simulink model "ES005A_TmplMonr"  (R2013b)
settings: Solver=FixedStepDiscrete  SolverMode=SingleTasking  StartTime=0.0  StopTime=1  FixedStep=0.002  RelTol=1e-3
undefined symbols (not defined in the file): ELECGLBPRM_STRTUPSTDI_CNT_U08, ELECGLBPRM_STRTUPSTTMPLMONININTESTSTRT_CNT_U08, IninFlt, RtFlt, SpiConf_SpiChannel_TmplMonrCh1, SpiConf_SpiChannel_TmplMonrCh2, SpiConf_SpiChannel_TmplMonrCh3, SpiConf_SpiSequence_TmplMonrSeq1, SpiConf_SpiSequence_TmplMonrSeq2, SpiConf_SpiSequence_TmplMonrSeq3, STD_HIGH, STD_LOW, TMPLMONRCFGREG1READVAL_CNT_U16, TMPLMONRCFGREG1WRVAL_CNT_U16, TMPLMONRSTSREG2READVAL_CNT_U16, TMPLMONRWDGMODKEYWORD1_CNT_U16, TMPLMONRWDGMODKEYWORD2_CNT_U16, TMPLMONRWDGMODKEYWORD3_CNT_U16, TrigReg1
libraries: simulink x12
(part 3 of 4)

== system ES005A_TmplMonr/TmplMonr/TmplMonrPer1/TMF Init Test/21/CopyRight1 ==

== system ES005A_TmplMonr/TmplMonr/TmplMonrPer1/TMF Init Test/21/Edge//Valid Cnts are NOT Correct ==
  note: NTCNR_0X040
      | Parameters:
      |     1 = 0000 0001 = Bit 0 = Fault Occured Between TmplMonrInitCntr =  10 ~ 11
      |     2 = 0000 0010 = Bit 1 = Fault Occured Between TmplMonrInitCntr = 13 (AND Gate Fault)
      |     4 = 0000 0100 = Bit 2 = Fault Occured Between TmplMonrInitCntr = 15 ~ 16
      |     8 = 0000 1000 = Bit 3 = Fault Occured at TmplMonrInitCntr            = 18  (POE Fault)
      |   16 = 0001 0000 = Bit 4 = Fault Occured at TmplMonrInitCntr            = 19 (WD_STATE Fault)
      |   32 = 0010 0000 = Bit 5 = Fault Occured at TmplMonrInitCntr            = 21 (Edge/Valid Write Fault)
      |   64 = 0100 0000 = Bit 6 = Fault Occured at TmplMonrInitCntr            = 53 (POE + Non-WD Fault)
      | 128 = 1000 0000 = Bit 7 = Fault Occured at TmplMonrInitCntr            = 53 (POE + WD Fault)
  Action Port : ActionPort  ActionType=then
  Bitwise Operator2 : simulink/Logic and Bit Operations/Bitwise Operator  logicop=OR  UseBitMask=off  NumInputPorts=2  BitMask=bin2dec('00001111')  BitMaskRealWorld=Stored Integer
  CopyRight1 : Subsystem  Description=|  mask(Copyright Information){none=on}
      | Copyright info block.                                               
      |                                                                     
      | Place copyright information at the top of every subsystem in design.
      mask prompts: none "No parameters"
      mask help: Place copyright information at the top of every subsystem in design.
      mask Display:
      | NxtrConf = 'Nexteer Confidential';
      | 
      | sys = bdroot; %handle for the current model ("system")
      | first = get_param(sys,'Created');
      | first = first(end-3:end);  %year is last four digits
      | 
      | last = get_param(sys,'LastModifiedDate');
      | if isempty(last)
      |     last = datestr(now,'yyyy');
      | else
      |     last = last(end-3:end);
      | end
      | 
      | if strcmp(first,last)
      |     fprintf('%s -- Copyright %s Nexteer',NxtrConf,first)
      | else
      |     fprintf('%s -- %s%s- %s Nexteer',NxtrConf,char(169),first,last)
      | end
  Data Store Read3 : DataStoreRead  DataStoreName=TmplMonrNtc40PrmByte  DataStoreElements=TmplMonrNtc40PrmByte
  Data Store Write1 : DataStoreWrite  DataStoreName=TmplMonrNtc40PrmByte
  NtcStInfo : Constant  Value=32  OutDataTypeStr=uint8
  wires:
  Bitwise Operator2/1 -> Data Store Write1/1
  Data Store Read3/1 -> Bitwise Operator2/1
  NtcStInfo/1 -> Bitwise Operator2/2

== system ES005A_TmplMonr/TmplMonr/TmplMonrPer1/TMF Init Test/21/Spi_ReadIB ==
  note: Read Buffer - Simulation Purpose Only
      |
      |
      |
      |                            00001011
  Channel : Inport
  Constant1 : Constant  Value=11  OutDataTypeStr=uint16
  CopyRight1 : Subsystem  Description=|  mask(Copyright Information){none=on}
      | Copyright info block.                                               
      |                                                                     
      | Place copyright information at the top of every subsystem in design.
      mask prompts: none "No parameters"
      mask help: Place copyright information at the top of every subsystem in design.
      mask Display:
      | NxtrConf = 'Nexteer Confidential';
      | 
      | sys = bdroot; %handle for the current model ("system")
      | first = get_param(sys,'Created');
      | first = first(end-3:end);  %year is last four digits
      | 
      | last = get_param(sys,'LastModifiedDate');
      | if isempty(last)
      |     last = datestr(now,'yyyy');
      | else
      |     last = last(end-3:end);
      | end
      | 
      | if strcmp(first,last)
      |     fprintf('%s -- Copyright %s Nexteer',NxtrConf,first)
      | else
      |     fprintf('%s -- %s%s- %s Nexteer',NxtrConf,char(169),first,last)
      | end
  Terminator : Terminator
  Rx : Outport
  wires:
  Constant1/1 -> Rx/1
  Channel/1 -> Terminator/1

== system ES005A_TmplMonr/TmplMonr/TmplMonrPer1/TMF Init Test/22-52/CopyRight1 ==

== system ES005A_TmplMonr/TmplMonr/TmplMonrPer1/TMF Init Test/53/CopyRight1 ==

== system ES005A_TmplMonr/TmplMonr/TmplMonrPer1/TMF Init Test/53/Fault Condition - WD Run Fault ==
  Action Port : ActionPort  ActionType=else
  CopyRight1 : Subsystem  Description=|  mask(Copyright Information){none=on}
      | Copyright info block.                                               
      |                                                                     
      | Place copyright information at the top of every subsystem in design.
      mask prompts: none "No parameters"
      mask help: Place copyright information at the top of every subsystem in design.
      mask Display:
      | NxtrConf = 'Nexteer Confidential';
      | 
      | sys = bdroot; %handle for the current model ("system")
      | first = get_param(sys,'Created');
      | first = first(end-3:end);  %year is last four digits
      | 
      | last = get_param(sys,'LastModifiedDate');
      | if isempty(last)
      |     last = datestr(now,'yyyy');
      | else
      |     last = last(end-3:end);
      | end
      | 
      | if strcmp(first,last)
      |     fprintf('%s -- Copyright %s Nexteer',NxtrConf,first)
      | else
      |     fprintf('%s -- %s%s- %s Nexteer',NxtrConf,char(169),first,last)
      | end
  Data Store Read1 : DataStoreRead  DataStoreName=TmplMonrSpiReadWrOrderFlg1
  If : If  IfExpression=u1 == 0
  Merge1 : Merge
  Merge2 : Merge
  "TmplMonrSpiReadWrOrderFlg1 = 0 (Read Cmd) " : Subsystem
  TmplMonrSpiReadWrOrderFlg1 = 1 (Read Buffer) : Subsystem
  TmplMonrInitCntr : Outport
  TmplMonrIninTestCmpl : Outport  Port=2
  wires:
  If/1 -> "TmplMonrSpiReadWrOrderFlg1 = 0 (Read Cmd) "/Action
  If/2 -> TmplMonrSpiReadWrOrderFlg1 = 1 (Read Buffer)/Action
  Data Store Read1/1 -> If/1
  Merge1/1 -> TmplMonrInitCntr/1
  "TmplMonrSpiReadWrOrderFlg1 = 0 (Read Cmd) "/1(TmplMonrIninCntr) -> Merge1/1
  TmplMonrSpiReadWrOrderFlg1 = 1 (Read Buffer)/1(TmplMonrIninCntr) -> Merge1/2
  "TmplMonrSpiReadWrOrderFlg1 = 0 (Read Cmd) "/2(TmplMonrIninTestCmpl) -> Merge2/1
  TmplMonrSpiReadWrOrderFlg1 = 1 (Read Buffer)/2(TmplMonrIninTestCmpl) -> Merge2/2
  Merge2/1 -> TmplMonrIninTestCmpl/1

== system ES005A_TmplMonr/TmplMonr/TmplMonrPer1/TMF Init Test/53/IoHwAb_GetGpioPwrOutpEnaFb ==
  CopyRight1 : Subsystem  Description=|  mask(Copyright Information){none=on}
      | Copyright info block.                                               
      |                                                                     
      | Place copyright information at the top of every subsystem in design.
      mask prompts: none "No parameters"
      mask help: Place copyright information at the top of every subsystem in design.
      mask Display:
      | NxtrConf = 'Nexteer Confidential';
      | 
      | sys = bdroot; %handle for the current model ("system")
      | first = get_param(sys,'Created');
      | first = first(end-3:end);  %year is last four digits
      | 
      | last = get_param(sys,'LastModifiedDate');
      | if isempty(last)
      |     last = datestr(now,'yyyy');
      | else
      |     last = last(end-3:end);
      | end
      | 
      | if strcmp(first,last)
      |     fprintf('%s -- Copyright %s Nexteer',NxtrConf,first)
      | else
      |     fprintf('%s -- %s%s- %s Nexteer',NxtrConf,char(169),first,last)
      | end
  Ground : Ground
  PinSt : Outport
  wires:
  Ground/1 -> PinSt/1

== system ES005A_TmplMonr/TmplMonr/TmplMonrPer1/TMF Init Test/53/Normal Condition ==
  Action Port : ActionPort  ActionType=then
  Constant1 : Constant  OutDataTypeStr=boolean
  Constant2 : Constant  OutDataTypeStr=uint8
  Constant3 : Constant  Value=0  OutDataTypeStr=boolean
  Constant4 : Constant  OutDataTypeStr=boolean
  CopyRight1 : Subsystem  Description=|  mask(Copyright Information){none=on}
      | Copyright info block.                                               
      |                                                                     
      | Place copyright information at the top of every subsystem in design.
      mask prompts: none "No parameters"
      mask help: Place copyright information at the top of every subsystem in design.
      mask Display:
      | NxtrConf = 'Nexteer Confidential';
      | 
      | sys = bdroot; %handle for the current model ("system")
      | first = get_param(sys,'Created');
      | first = first(end-3:end);  %year is last four digits
      | 
      | last = get_param(sys,'LastModifiedDate');
      | if isempty(last)
      |     last = datestr(now,'yyyy');
      | else
      |     last = last(end-3:end);
      | end
      | 
      | if strcmp(first,last)
      |     fprintf('%s -- Copyright %s Nexteer',NxtrConf,first)
      | else
      |     fprintf('%s -- %s%s- %s Nexteer',NxtrConf,char(169),first,last)
      | end
  Data Store Write : DataStoreWrite  DataStoreName=TmplMonrSpiReadWrOrderFlg1
  Data Store Write2 : DataStoreWrite  DataStoreName=TmplMonrIninTestCmplFlg
      settings: AttributesFormatString=%<Name>
  TmplMonrIninCntr : Outport
  TmplMonrIninTestCmpl : Outport  Port=2
  wires:
  Constant2/1 -> TmplMonrIninCntr/1
  Constant1/1 -> TmplMonrIninTestCmpl/1
  Constant3/1 -> Data Store Write/1
  Constant4/1 -> Data Store Write2/1

== system ES005A_TmplMonr/TmplMonr/TmplMonrPer1/TMF Init Test/53/Set NTC 0x040 Note: Run last ==
  note: NTCNR_0X040
      | Parameters:
      |     1 = 0000 0001 = Bit 0 = Fault Occured Between TmplMonrInitCntr =  10 ~ 11
      |     2 = 0000 0010 = Bit 1 = Fault Occured Between TmplMonrInitCntr = 13 (AND Gate Fault)
      |     4 = 0000 0100 = Bit 2 = Fault Occured Between TmplMonrInitCntr = 15 ~ 16
      |     8 = 0000 1000 = Bit 3 = Fault Occured at TmplMonrInitCntr            = 18  (POE Fault)
      |   16 = 0001 0000 = Bit 4 = Fault Occured at TmplMonrInitCntr            = 19 (WD_STATE Fault)
      |   32 = 0010 0000 = Bit 5 = Fault Occured at TmplMonrInitCntr            = 21 (Edge/Valid Write Fault)
      |   64 = 0100 0000 = Bit 6 = Fault Occured at TmplMonrInitCntr            = 53 (POE + Non-WD Fault)
      | 128 = 1000 0000 = Bit 7 = Fault Occured at TmplMonrInitCntr            = 53 (POE + WD Fault)
  Data Store Read2 : DataStoreRead  DataStoreName=TmplMonrNtc40PrmByte  DataStoreElements=TmplMonrNtc40PrmByte
  FAILED = 1 : Subsystem
  If : If  IfExpression=u1 == 0
  PASSED = 0 : Subsystem
  wires:
  Data Store Read2/1 -> If/1, FAILED = 1/1(NtcStInfo)
  If/1 -> PASSED = 0/Action
  If/2 -> FAILED = 1/Action

== system ES005A_TmplMonr/TmplMonr/TmplMonrPer1/TMF Init Test/Default/CopyRight1 ==

== system ES005A_TmplMonr/TmplMonr/TmplMonrPer1/TMF Init Test/IoHwAb_SetGpioTmplMonrWdg/CopyRight1 ==

== system ES005A_TmplMonr/TmplMonr/TmplMonrPer1/TMF Init Test/IoHwAb_SetGpioTmplMonrWdg/IoHwAb_SetGpioTmplMonrWdg ==
  PinSt : Inport
  CopyRight1 : Subsystem  Description=|  mask(Copyright Information){none=on}
      | Copyright info block.                                               
      |                                                                     
      | Place copyright information at the top of every subsystem in design.
      mask prompts: none "No parameters"
      mask help: Place copyright information at the top of every subsystem in design.
      mask Display:
      | NxtrConf = 'Nexteer Confidential';
      | 
      | sys = bdroot; %handle for the current model ("system")
      | first = get_param(sys,'Created');
      | first = first(end-3:end);  %year is last four digits
      | 
      | last = get_param(sys,'LastModifiedDate');
      | if isempty(last)
      |     last = datestr(now,'yyyy');
      | else
      |     last = last(end-3:end);
      | end
      | 
      | if strcmp(first,last)
      |     fprintf('%s -- Copyright %s Nexteer',NxtrConf,first)
      | else
      |     fprintf('%s -- %s%s- %s Nexteer',NxtrConf,char(169),first,last)
      | end
  Terminator : Terminator
  wires:
  PinSt/1 -> Terminator/1

== system ES005A_TmplMonr/TmplMonr/TmplMonrPer1/TMF Init Test/nError Signal Control/CopyRight1 ==

== system ES005A_TmplMonr/TmplMonr/TmplMonrPer1/TMF Init Test/nError Signal Control/CtrlErrOut  ==
  PinSt_ArgIn : Inport
  TrigReg_ArgIn : Inport  Port=2
  CopyRight1 : Subsystem  Description=|  mask(Copyright Information){none=on}
      | Copyright info block.                                               
      |                                                                     
      | Place copyright information at the top of every subsystem in design.
      mask prompts: none "No parameters"
      mask help: Place copyright information at the top of every subsystem in design.
      mask Display:
      | NxtrConf = 'Nexteer Confidential';
      | 
      | sys = bdroot; %handle for the current model ("system")
      | first = get_param(sys,'Created');
      | first = first(end-3:end);  %year is last four digits
      | 
      | last = get_param(sys,'LastModifiedDate');
      | if isempty(last)
      |     last = datestr(now,'yyyy');
      | else
      |     last = last(end-3:end);
      | end
      | 
      | if strcmp(first,last)
      |     fprintf('%s -- Copyright %s Nexteer',NxtrConf,first)
      | else
      |     fprintf('%s -- %s%s- %s Nexteer',NxtrConf,char(169),first,last)
      | end
  Terminator : Terminator
  Terminator1 : Terminator
  wires:
  PinSt_ArgIn/1 -> Terminator/1
  TrigReg_ArgIn/1 -> Terminator1/1

== system ES005A_TmplMonr/TmplMonr/TmplMonrPer1/TMF Run/Fault Condition - WD Run Fault/CopyRight1 ==

== system ES005A_TmplMonr/TmplMonr/TmplMonrPer1/TMF Run/Fault Condition - WD Run Fault/TmplMonrSpiReadWrOrderFlg2 = 0 (Read Cmd)  ==
  note: Read Cmd: Watchdog State - 00010 0 0 00000000
  Action Port : ActionPort  ActionType=then
  Call_Spi_AsyncTransmit : Subsystem
  Constant1 : Constant  OutDataTypeStr=boolean
  Constant5 : Constant  Value=SpiConf_SpiSequence_TmplMonrSeq1  OutDataTypeStr=uint8
  Constant6 : Constant  Value=SpiConf_SpiChannel_TmplMonrCh1  OutDataTypeStr=uint8
  Constant7 : Constant  Value=TMPLMONRSTSREG2READVAL_CNT_U16  OutDataTypeStr=uint16
  CopyRight1 : Subsystem  Description=|  mask(Copyright Information){none=on}
      | Copyright info block.                                               
      |                                                                     
      | Place copyright information at the top of every subsystem in design.
      mask prompts: none "No parameters"
      mask help: Place copyright information at the top of every subsystem in design.
      mask Display:
      | NxtrConf = 'Nexteer Confidential';
      | 
      | sys = bdroot; %handle for the current model ("system")
      | first = get_param(sys,'Created');
      | first = first(end-3:end);  %year is last four digits
      | 
      | last = get_param(sys,'LastModifiedDate');
      | if isempty(last)
      |     last = datestr(now,'yyyy');
      | else
      |     last = last(end-3:end);
      | end
      | 
      | if strcmp(first,last)
      |     fprintf('%s -- Copyright %s Nexteer',NxtrConf,first)
      | else
      |     fprintf('%s -- %s%s- %s Nexteer',NxtrConf,char(169),first,last)
      | end
  Data Store Write : DataStoreWrite  DataStoreName=TmplMonrSpiReadWrOrderFlg2
  Spi_WriteIB : Subsystem
  wires:
  Constant1/1 -> Data Store Write/1
  Constant5/1 -> Call_Spi_AsyncTransmit/1(Sequence)
  Constant6/1 -> Spi_WriteIB/1(Channel)
  Constant7/1 -> Spi_WriteIB/2(DataBufferPtr)

== system ES005A_TmplMonr/TmplMonr/TmplMonrPer1/TMF Run/Fault Condition - WD Run Fault/TmplMonrSpiReadWrOrderFlg2 = 1 (Read Buffer) ==
  note: Read Buffer: Watchdog State
  Action Port : ActionPort  ActionType=else
  Bitwise Operator1 : simulink/Logic and Bit Operations/Bitwise Operator  logicop=AND  UseBitMask=on  BitMask=bin2dec('00000111')  BitMaskRealWorld=Stored Integer
  Constant1 : Constant  Value=0  OutDataTypeStr=boolean
  Constant4 : Constant  Value=SpiConf_SpiChannel_TmplMonrCh1  OutDataTypeStr=uint8
  CopyRight1 : Subsystem  Description=|  mask(Copyright Information){none=on}
      | Copyright info block.                                               
      |                                                                     
      | Place copyright information at the top of every subsystem in design.
      mask prompts: none "No parameters"
      mask help: Place copyright information at the top of every subsystem in design.
      mask Display:
      | NxtrConf = 'Nexteer Confidential';
      | 
      | sys = bdroot; %handle for the current model ("system")
      | first = get_param(sys,'Created');
      | first = first(end-3:end);  %year is last four digits
      | 
      | last = get_param(sys,'LastModifiedDate');
      | if isempty(last)
      |     last = datestr(now,'yyyy');
      | else
      |     last = last(end-3:end);
      | end
      | 
      | if strcmp(first,last)
      |     fprintf('%s -- Copyright %s Nexteer',NxtrConf,first)
      | else
      |     fprintf('%s -- %s%s- %s Nexteer',NxtrConf,char(169),first,last)
      | end
  Data Store Write : DataStoreWrite  DataStoreName=TmplMonrSpiReadWrOrderFlg2
  If : If  IfExpression=u1 ~= 7
  Spi_ReadIB : Subsystem
  WD_STATE = NOT Watchdog (~7) : Subsystem
  WD_STATE = Watchdog (7) : Subsystem
  wires:
  Constant1/1 -> Data Store Write/1
  Bitwise Operator1/1 -> If/1
  If/1 -> WD_STATE = NOT Watchdog (~7)/Action
  If/2 -> WD_STATE = Watchdog (7)/Action
  Constant4/1 -> Spi_ReadIB/1(Channel)
  Spi_ReadIB/1(Rx) -> Bitwise Operator1/1

== system ES005A_TmplMonr/TmplMonr/TmplMonrPer1/TMF Run/IoHwAb_GetGpioPwrOutpEnaFb/CopyRight1 ==

== system ES005A_TmplMonr/TmplMonr/TmplMonrPer1/TMF Run/IoHwAb_SetGpioTmplMonrWdg1/CopyRight1 ==

== system ES005A_TmplMonr/TmplMonr/TmplMonrPer1/TMF Run/Normal Condition/CopyRight1 ==

== system ES005A_TmplMonr/TmplMonr/TmplMonrPer1/TMF Run/Normal Condition/SetNtcSts ==
  note: Note:
      |
      | - "ISO Fault Debounce Design" Simulink block intent to use here for Simulation purpose only. Do not Code this block
  NtcNr : Inport
  NtcStInfo : Inport  Port=2
  NtcSts : Inport  Port=3  OutDataTypeStr=uint8
  DebStep : Inport  Port=4
  CopyRight2 : Subsystem  Description=|  mask(Copyright Information){none=on}
      | Copyright info block.                                               
      |                                                                     
      | Place copyright information at the top of every subsystem in design.
      mask prompts: none "No parameters"
      mask help: Place copyright information at the top of every subsystem in design.
      mask Display:
      | NxtrConf = 'Nexteer Confidential';
      | 
      | sys = bdroot; %handle for the current model ("system")
      | first = get_param(sys,'Created');
      | first = first(end-3:end);  %year is last four digits
      | 
      | last = get_param(sys,'LastModifiedDate');
      | if isempty(last)
      |     last = datestr(now,'yyyy');
      | else
      |     last = last(end-3:end);
      | end
      | 
      | if strcmp(first,last)
      |     fprintf('%s -- Copyright %s Nexteer',NxtrConf,first)
      | else
      |     fprintf('%s -- %s%s- %s Nexteer',NxtrConf,char(169),first,last)
      | end
  Ground : Ground
  ISO Fault Debounce Design : Stateflow chart  TreatAsAtomicUnit=on
      settings: AttributesFormatString=|
      | Simulation Purpose Only.
      | Do Not Code this block
      | Diagnostic Manager Owns this requirement
  Scope1 : Scope  NumInputPorts=3
      settings: YMin=-5~-5~-5  YMax=5~5~5  SaveName=ScopeData5
  Terminator : Terminator
  Terminator1 : Terminator
  wires:
  NtcStInfo/1 -> Terminator1/1
  NtcNr/1 -> Terminator/1
  NtcSts/1 -> ISO Fault Debounce Design/1(NtcSts), Scope1/1
  DebStep/1 -> ISO Fault Debounce Design/2(DebStep), Scope1/2
  ISO Fault Debounce Design/1(Qualifier) -> Scope1/3
  Ground/1 -> ISO Fault Debounce Design/3(SvcClr)

== system ES005A_TmplMonr/TmplMonr/TmplMonrPer2/Subsystem/IoHwAb_SetGpioSysFlt2A/CopyRight1 ==

== system ES005A_TmplMonr/TmplMonr/TmplMonrPer2/Subsystem/IoHwAb_SetGpioSysFlt2B/CopyRight1 ==

== system ES005A_TmplMonr/TmplMonr/TmplMonrPer1/TMF Init Test/0/Watchdog Mode Key: Word1/Call_Spi_AsyncTransmit ==
  Sequence : Inport
  CopyRight1 : Subsystem  Description=|  mask(Copyright Information){none=on}
      | Copyright info block.                                               
      |                                                                     
      | Place copyright information at the top of every subsystem in design.
      mask prompts: none "No parameters"
      mask help: Place copyright information at the top of every subsystem in design.
      mask Display:
      | NxtrConf = 'Nexteer Confidential';
      | 
      | sys = bdroot; %handle for the current model ("system")
      | first = get_param(sys,'Created');
      | first = first(end-3:end);  %year is last four digits
      | 
      | last = get_param(sys,'LastModifiedDate');
      | if isempty(last)
      |     last = datestr(now,'yyyy');
      | else
      |     last = last(end-3:end);
      | end
      | 
      | if strcmp(first,last)
      |     fprintf('%s -- Copyright %s Nexteer',NxtrConf,first)
      | else
      |     fprintf('%s -- %s%s- %s Nexteer',NxtrConf,char(169),first,last)
      | end
  Terminator : Terminator
  wires:
  Sequence/1 -> Terminator/1

== system ES005A_TmplMonr/TmplMonr/TmplMonrPer1/TMF Init Test/0/Watchdog Mode Key: Word1/CopyRight1 ==

== system ES005A_TmplMonr/TmplMonr/TmplMonrPer1/TMF Init Test/0/Watchdog Mode Key: Word1/Spi_WriteIB ==
  Channel : Inport
  DataBufferPtr : Inport  Port=2
  CopyRight1 : Subsystem  Description=|  mask(Copyright Information){none=on}
      | Copyright info block.                                               
      |                                                                     
      | Place copyright information at the top of every subsystem in design.
      mask prompts: none "No parameters"
      mask help: Place copyright information at the top of every subsystem in design.
      mask Display:
      | NxtrConf = 'Nexteer Confidential';
      | 
      | sys = bdroot; %handle for the current model ("system")
      | first = get_param(sys,'Created');
      | first = first(end-3:end);  %year is last four digits
      | 
      | last = get_param(sys,'LastModifiedDate');
      | if isempty(last)
      |     last = datestr(now,'yyyy');
      | else
      |     last = last(end-3:end);
      | end
      | 
      | if strcmp(first,last)
      |     fprintf('%s -- Copyright %s Nexteer',NxtrConf,first)
      | else
      |     fprintf('%s -- %s%s- %s Nexteer',NxtrConf,char(169),first,last)
      | end
  Terminator : Terminator
  Terminator1 : Terminator
  wires:
  Channel/1 -> Terminator/1
  DataBufferPtr/1 -> Terminator1/1

== system ES005A_TmplMonr/TmplMonr/TmplMonrPer1/TMF Init Test/0/Watchdog Mode Key: Word2/Call_Spi_AsyncTransmit ==
  Sequence : Inport
  CopyRight1 : Subsystem  Description=|  mask(Copyright Information){none=on}
      | Copyright info block.                                               
      |                                                                     
      | Place copyright information at the top of every subsystem in design.
      mask prompts: none "No parameters"
      mask help: Place copyright information at the top of every subsystem in design.
      mask Display:
      | NxtrConf = 'Nexteer Confidential';
      | 
      | sys = bdroot; %handle for the current model ("system")
      | first = get_param(sys,'Created');
      | first = first(end-3:end);  %year is last four digits
      | 
      | last = get_param(sys,'LastModifiedDate');
      | if isempty(last)
      |     last = datestr(now,'yyyy');
      | else
      |     last = last(end-3:end);
      | end
      | 
      | if strcmp(first,last)
      |     fprintf('%s -- Copyright %s Nexteer',NxtrConf,first)
      | else
      |     fprintf('%s -- %s%s- %s Nexteer',NxtrConf,char(169),first,last)
      | end
  Terminator : Terminator
  wires:
  Sequence/1 -> Terminator/1

== system ES005A_TmplMonr/TmplMonr/TmplMonrPer1/TMF Init Test/0/Watchdog Mode Key: Word2/CopyRight1 ==

== system ES005A_TmplMonr/TmplMonr/TmplMonrPer1/TMF Init Test/0/Watchdog Mode Key: Word2/Spi_WriteIB ==
  Channel : Inport
  DataBufferPtr : Inport  Port=2
  CopyRight1 : Subsystem  Description=|  mask(Copyright Information){none=on}
      | Copyright info block.                                               
      |                                                                     
      | Place copyright information at the top of every subsystem in design.
      mask prompts: none "No parameters"
      mask help: Place copyright information at the top of every subsystem in design.
      mask Display:
      | NxtrConf = 'Nexteer Confidential';
      | 
      | sys = bdroot; %handle for the current model ("system")
      | first = get_param(sys,'Created');
      | first = first(end-3:end);  %year is last four digits
      | 
      | last = get_param(sys,'LastModifiedDate');
      | if isempty(last)
      |     last = datestr(now,'yyyy');
      | else
      |     last = last(end-3:end);
      | end
      | 
      | if strcmp(first,last)
      |     fprintf('%s -- Copyright %s Nexteer',NxtrConf,first)
      | else
      |     fprintf('%s -- %s%s- %s Nexteer',NxtrConf,char(169),first,last)
      | end
  Terminator : Terminator
  Terminator1 : Terminator
  wires:
  Channel/1 -> Terminator/1
  DataBufferPtr/1 -> Terminator1/1

== system ES005A_TmplMonr/TmplMonr/TmplMonrPer1/TMF Init Test/0/Watchdog Mode Key: Word3/Call_Spi_AsyncTransmit ==
  Sequence : Inport
  CopyRight1 : Subsystem  Description=|  mask(Copyright Information){none=on}
      | Copyright info block.                                               
      |                                                                     
      | Place copyright information at the top of every subsystem in design.
      mask prompts: none "No parameters"
      mask help: Place copyright information at the top of every subsystem in design.
      mask Display:
      | NxtrConf = 'Nexteer Confidential';
      | 
      | sys = bdroot; %handle for the current model ("system")
      | first = get_param(sys,'Created');
      | first = first(end-3:end);  %year is last four digits
      | 
      | last = get_param(sys,'LastModifiedDate');
      | if isempty(last)
      |     last = datestr(now,'yyyy');
      | else
      |     last = last(end-3:end);
      | end
      | 
      | if strcmp(first,last)
      |     fprintf('%s -- Copyright %s Nexteer',NxtrConf,first)
      | else
      |     fprintf('%s -- %s%s- %s Nexteer',NxtrConf,char(169),first,last)
      | end
  Terminator : Terminator
  wires:
  Sequence/1 -> Terminator/1

== system ES005A_TmplMonr/TmplMonr/TmplMonrPer1/TMF Init Test/0/Watchdog Mode Key: Word3/CopyRight1 ==

== system ES005A_TmplMonr/TmplMonr/TmplMonrPer1/TMF Init Test/0/Watchdog Mode Key: Word3/Spi_WriteIB ==
  Channel : Inport
  DataBufferPtr : Inport  Port=2
  CopyRight1 : Subsystem  Description=|  mask(Copyright Information){none=on}
      | Copyright info block.                                               
      |                                                                     
      | Place copyright information at the top of every subsystem in design.
      mask prompts: none "No parameters"
      mask help: Place copyright information at the top of every subsystem in design.
      mask Display:
      | NxtrConf = 'Nexteer Confidential';
      | 
      | sys = bdroot; %handle for the current model ("system")
      | first = get_param(sys,'Created');
      | first = first(end-3:end);  %year is last four digits
      | 
      | last = get_param(sys,'LastModifiedDate');
      | if isempty(last)
      |     last = datestr(now,'yyyy');
      | else
      |     last = last(end-3:end);
      | end
      | 
      | if strcmp(first,last)
      |     fprintf('%s -- Copyright %s Nexteer',NxtrConf,first)
      | else
      |     fprintf('%s -- %s%s- %s Nexteer',NxtrConf,char(169),first,last)
      | end
  Terminator : Terminator
  Terminator1 : Terminator
  wires:
  Channel/1 -> Terminator/1
  DataBufferPtr/1 -> Terminator1/1

== system ES005A_TmplMonr/TmplMonr/TmplMonrPer1/TMF Init Test/10-11, 15-17/IoHwAb_GetGpioPwrOutpEnaFb1/CopyRight1 ==

== system ES005A_TmplMonr/TmplMonr/TmplMonrPer1/TMF Init Test/10-11, 15-17/IoHwAb_GetGpioPwrOutpEnaFb1/Fault Condition - WD Signal ==
  note: NTCNR_0X040
      | Parameters:
      |     1 = 0000 0001 = Bit 0 = Fault Occured Between TmplMonrInitCntr =  10 ~ 11
      |     2 = 0000 0010 = Bit 1 = Fault Occured Between TmplMonrInitCntr = 13 (AND Gate Fault)
      |     4 = 0000 0100 = Bit 2 = Fault Occured Between TmplMonrInitCntr = 15 ~ 16
      |     8 = 0000 1000 = Bit 3 = Fault Occured at TmplMonrInitCntr            = 18  (POE Fault)
      |   16 = 0001 0000 = Bit 4 = Fault Occured at TmplMonrInitCntr            = 19 (WD_STATE Fault)
      |   32 = 0010 0000 = Bit 5 = Fault Occured at TmplMonrInitCntr            = 21 (Edge/Valid Write Fault)
      |   64 = 0100 0000 = Bit 6 = Fault Occured at TmplMonrInitCntr            = 53 (POE + Non-WD Fault)
      | 128 = 1000 0000 = Bit 7 = Fault Occured at TmplMonrInitCntr            = 53 (POE + WD Fault)
  Action Port : ActionPort  ActionType=then
  Bitwise Operator2 : simulink/Logic and Bit Operations/Bitwise Operator  logicop=OR  UseBitMask=off  NumInputPorts=2  BitMask=bin2dec('00001111')  BitMaskRealWorld=Stored Integer
  CopyRight1 : Subsystem  Description=|  mask(Copyright Information){none=on}
      | Copyright info block.                                               
      |                                                                     
      | Place copyright information at the top of every subsystem in design.
      mask prompts: none "No parameters"
      mask help: Place copyright information at the top of every subsystem in design.
      mask Display:
      | NxtrConf = 'Nexteer Confidential';
      | 
      | sys = bdroot; %handle for the current model ("system")
      | first = get_param(sys,'Created');
      | first = first(end-3:end);  %year is last four digits
      | 
      | last = get_param(sys,'LastModifiedDate');
      | if isempty(last)
      |     last = datestr(now,'yyyy');
      | else
      |     last = last(end-3:end);
      | end
      | 
      | if strcmp(first,last)
      |     fprintf('%s -- Copyright %s Nexteer',NxtrConf,first)
      | else
      |     fprintf('%s -- %s%s- %s Nexteer',NxtrConf,char(169),first,last)
      | end
  Data Store Read1 : DataStoreRead  DataStoreName=TmplMonrIninCntr
  Data Store Read3 : DataStoreRead  DataStoreName=TmplMonrNtc40PrmByte  DataStoreElements=TmplMonrNtc40PrmByte
  Data Store Write1 : DataStoreWrite  DataStoreName=TmplMonrNtc40PrmByte
  NtcStInfo1 : Constant  RequirementInfo={'linktype_rmi_doors' '0000c46a (/ESG Group/FDD Module Requirements/EA4 Specific/ES005A_TmplMonr)' '#ES005A_172' 'true' 'REQ: ES005A_172' '' } %GIDa_8076c81f_319b_4d5e_9856_dc13330ba5d4  Value=4  OutDataTypeStr=uint8
  NtcStInfo2 : Constant  RequirementInfo={'linktype_rmi_doors' '0000c46a (/ESG Group/FDD Module Requirements/EA4 Specific/ES005A_TmplMonr)' '#ES005A_163' 'true' 'REQ: ES005A_163' '' } %GIDa_4ff45b97_9198_4bb3_bfa4_37df695f7f6b  OutDataTypeStr=uint8
  Switch : Switch  Criteria=u2 > Threshold  Threshold=14
  wires:
  NtcStInfo2/1 -> Switch/3
  NtcStInfo1/1 -> Switch/1
  Data Store Read1/1 -> Switch/2
  Bitwise Operator2/1 -> Data Store Write1/1
  Data Store Read3/1 -> Bitwise Operator2/1
  Switch/1 -> Bitwise Operator2/2

== system ES005A_TmplMonr/TmplMonr/TmplMonrPer1/TMF Init Test/10-11, 15-17/IoHwAb_GetGpioPwrOutpEnaFb1/IoHwAb_GetGpioPwrOutpEnaFb ==
  CopyRight1 : Subsystem  Description=|  mask(Copyright Information){none=on}
      | Copyright info block.                                               
      |                                                                     
      | Place copyright information at the top of every subsystem in design.
      mask prompts: none "No parameters"
      mask help: Place copyright information at the top of every subsystem in design.
      mask Display:
      | NxtrConf = 'Nexteer Confidential';
      | 
      | sys = bdroot; %handle for the current model ("system")
      | first = get_param(sys,'Created');
      | first = first(end-3:end);  %year is last four digits
      | 
      | last = get_param(sys,'LastModifiedDate');
      | if isempty(last)
      |     last = datestr(now,'yyyy');
      | else
      |     last = last(end-3:end);
      | end
      | 
      | if strcmp(first,last)
      |     fprintf('%s -- Copyright %s Nexteer',NxtrConf,first)
      | else
      |     fprintf('%s -- %s%s- %s Nexteer',NxtrConf,char(169),first,last)
      | end
  Ground : Ground
  PinSt : Outport
  wires:
  Ground/1 -> PinSt/1

== system ES005A_TmplMonr/TmplMonr/TmplMonrPer1/TMF Init Test/13/Fault Condition - AND Gate/CopyRight1 ==

== system ES005A_TmplMonr/TmplMonr/TmplMonrPer1/TMF Init Test/13/IoHwAb_GetGpioPwrOutpEnaFb/CopyRight1 ==

== system ES005A_TmplMonr/TmplMonr/TmplMonrPer1/TMF Init Test/18/Call_Spi_AsyncTransmit/CopyRight1 ==

== system ES005A_TmplMonr/TmplMonr/TmplMonrPer1/TMF Init Test/18/Fault Condition - WD/CopyRight1 ==

== system ES005A_TmplMonr/TmplMonr/TmplMonrPer1/TMF Init Test/18/IoHwAb_GetGpioPwrOutpEnaFb/CopyRight1 ==

== system ES005A_TmplMonr/TmplMonr/TmplMonrPer1/TMF Init Test/18/Spi_WriteIB/CopyRight1 ==

== system ES005A_TmplMonr/TmplMonr/TmplMonrPer1/TMF Init Test/19/Spi_ReadIB/CopyRight1 ==

== system ES005A_TmplMonr/TmplMonr/TmplMonrPer1/TMF Init Test/19/WD_STATE = 0 ~ 2, 7/CopyRight1 ==

== system ES005A_TmplMonr/TmplMonr/TmplMonrPer1/TMF Init Test/19/WD_STATE = 0 ~ 2, 7/Jump to Stage 53 ==
  Action Port : ActionPort  ActionType=else
  Bitwise Operator2 : simulink/Logic and Bit Operations/Bitwise Operator  logicop=OR  UseBitMask=off  NumInputPorts=2  BitMask=bin2dec('00001111')  BitMaskRealWorld=Stored Integer
  Constant1 : Constant  Value=53  OutDataTypeStr=uint8
  CopyRight1 : Subsystem  Description=|  mask(Copyright Information){none=on}
      | Copyright info block.                                               
      |                                                                     
      | Place copyright information at the top of every subsystem in design.
      mask prompts: none "No parameters"
      mask help: Place copyright information at the top of every subsystem in design.
      mask Display:
      | NxtrConf = 'Nexteer Confidential';
      | 
      | sys = bdroot; %handle for the current model ("system")
      | first = get_param(sys,'Created');
      | first = first(end-3:end);  %year is last four digits
      | 
      | last = get_param(sys,'LastModifiedDate');
      | if isempty(last)
      |     last = datestr(now,'yyyy');
      | else
      |     last = last(end-3:end);
      | end
      | 
      | if strcmp(first,last)
      |     fprintf('%s -- Copyright %s Nexteer',NxtrConf,first)
      | else
      |     fprintf('%s -- %s%s- %s Nexteer',NxtrConf,char(169),first,last)
      | end
  Data Store Read3 : DataStoreRead  DataStoreName=TmplMonrNtc40PrmByte  DataStoreElements=TmplMonrNtc40PrmByte
  Data Store Write1 : DataStoreWrite  DataStoreName=TmplMonrIninCntr
  Data Store Write2 : DataStoreWrite  DataStoreName=TmplMonrNtc40PrmByte
  NtcStInfo : Constant  Value=16  OutDataTypeStr=uint8
  wires:
  Constant1/1 -> Data Store Write1/1
  Bitwise Operator2/1 -> Data Store Write2/1
  Data Store Read3/1 -> Bitwise Operator2/1
  NtcStInfo/1 -> Bitwise Operator2/2

== system ES005A_TmplMonr/TmplMonr/TmplMonrPer1/TMF Init Test/19/WD_STATE = 0 ~ 2, 7/WD RESTART - Two Retry ==
  Action Port : ActionPort  ActionType=then
  Add : Sum  Inputs=++|
  Constant1 : Constant  OutDataTypeStr=uint8
  CopyRight1 : Subsystem  Description=|  mask(Copyright Information){none=on}
      | Copyright info block.                                               
      |                                                                     
      | Place copyright information at the top of every subsystem in design.
      mask prompts: none "No parameters"
      mask help: Place copyright information at the top of every subsystem in design.
      mask Display:
      | NxtrConf = 'Nexteer Confidential';
      | 
      | sys = bdroot; %handle for the current model ("system")
      | first = get_param(sys,'Created');
      | first = first(end-3:end);  %year is last four digits
      | 
      | last = get_param(sys,'LastModifiedDate');
      | if isempty(last)
      |     last = datestr(now,'yyyy');
      | else
      |     last = last(end-3:end);
      | end
      | 
      | if strcmp(first,last)
      |     fprintf('%s -- Copyright %s Nexteer',NxtrConf,first)
      | else
      |     fprintf('%s -- %s%s- %s Nexteer',NxtrConf,char(169),first,last)
      | end
  Data Store Read1 : DataStoreRead  DataStoreName=TmplMonrWdgRstrtCnt
  Data Store Write : DataStoreWrite  DataStoreName=TmplMonrWdgRstrtCnt
  Data Store Write1 : DataStoreWrite  DataStoreName=TmplMonrIninCntr
  Data Store Write4 : DataStoreWrite  DataStoreName=TmplMonrNtc40PrmByte
  constant : Constant  Value=0  OutDataTypeStr=uint8
  constant1 : Constant  Value=0  OutDataTypeStr=uint8
  wires:
  constant/1 -> Data Store Write1/1
  constant1/1 -> Data Store Write4/1
  Constant1/1 -> Add/2
  Add/1 -> Data Store Write/1
  Data Store Read1/1 -> Add/1

== system ES005A_TmplMonr/TmplMonr/TmplMonrPer1/TMF Init Test/19/WD_STATE = 3 ~ 6/Call_Spi_AsyncTransmit ==
  Sequence : Inport
  CopyRight1 : Subsystem  Description=|  mask(Copyright Information){none=on}
      | Copyright info block.                                               
      |                                                                     
      | Place copyright information at the top of every subsystem in design.
      mask prompts: none "No parameters"
      mask help: Place copyright information at the top of every subsystem in design.
      mask Display:
      | NxtrConf = 'Nexteer Confidential';
      | 
      | sys = bdroot; %handle for the current model ("system")
      | first = get_param(sys,'Created');
      | first = first(end-3:end);  %year is last four digits
      | 
      | last = get_param(sys,'LastModifiedDate');
      | if isempty(last)
      |     last = datestr(now,'yyyy');
      | else
      |     last = last(end-3:end);
      | end
      | 
      | if strcmp(first,last)
      |     fprintf('%s -- Copyright %s Nexteer',NxtrConf,first)
      | else
      |     fprintf('%s -- %s%s- %s Nexteer',NxtrConf,char(169),first,last)
      | end
  Terminator : Terminator
  wires:
  Sequence/1 -> Terminator/1

== system ES005A_TmplMonr/TmplMonr/TmplMonrPer1/TMF Init Test/19/WD_STATE = 3 ~ 6/CopyRight1 ==

== system ES005A_TmplMonr/TmplMonr/TmplMonrPer1/TMF Init Test/19/WD_STATE = 3 ~ 6/Spi_WriteIB ==
  Channel : Inport
  DataBufferPtr : Inport  Port=2
  CopyRight1 : Subsystem  Description=|  mask(Copyright Information){none=on}
      | Copyright info block.                                               
      |                                                                     
      | Place copyright information at the top of every subsystem in design.
      mask prompts: none "No parameters"
      mask help: Place copyright information at the top of every subsystem in design.
      mask Display:
      | NxtrConf = 'Nexteer Confidential';
      | 
      | sys = bdroot; %handle for the current model ("system")
      | first = get_param(sys,'Created');
      | first = first(end-3:end);  %year is last four digits
      | 
      | last = get_param(sys,'LastModifiedDate');
      | if isempty(last)
      |     last = datestr(now,'yyyy');
      | else
      |     last = last(end-3:end);
      | end
      | 
      | if strcmp(first,last)
      |     fprintf('%s -- Copyright %s Nexteer',NxtrConf,first)
      | else
      |     fprintf('%s -- %s%s- %s Nexteer',NxtrConf,char(169),first,last)
      | end
  Terminator : Terminator
  Terminator1 : Terminator
  wires:
  Channel/1 -> Terminator/1
  DataBufferPtr/1 -> Terminator1/1

== system ES005A_TmplMonr/TmplMonr/TmplMonrPer1/TMF Init Test/20/Call_Spi_AsyncTransmit/CopyRight1 ==

== system ES005A_TmplMonr/TmplMonr/TmplMonrPer1/TMF Init Test/20/Spi_WriteIB/CopyRight1 ==

== system ES005A_TmplMonr/TmplMonr/TmplMonrPer1/TMF Init Test/21/Edge//Valid Cnts are NOT Correct/CopyRight1 ==

== system ES005A_TmplMonr/TmplMonr/TmplMonrPer1/TMF Init Test/21/Spi_ReadIB/CopyRight1 ==

== system ES005A_TmplMonr/TmplMonr/TmplMonrPer1/TMF Init Test/53/Fault Condition - WD Run Fault/CopyRight1 ==

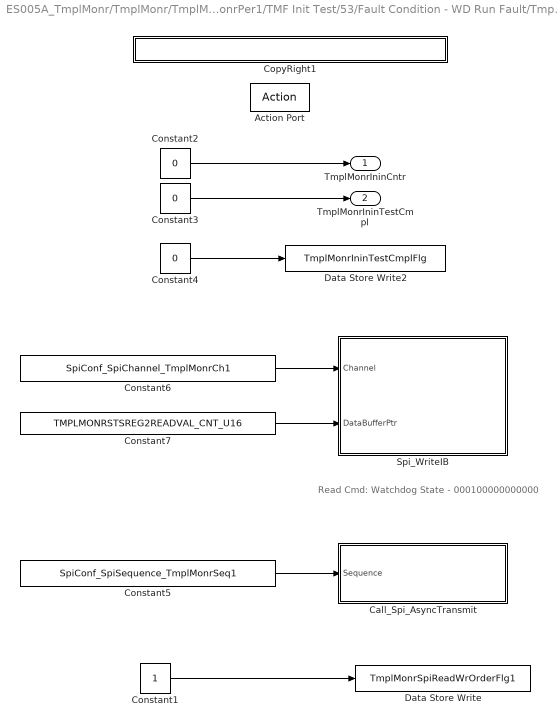
== system ES005A_TmplMonr/TmplMonr/TmplMonrPer1/TMF Init Test/53/Fault Condition - WD Run Fault/TmplMonrSpiReadWrOrderFlg1 = 0 (Read Cmd)  ==
  note: Read Cmd: Watchdog State - 000100000000000
  Action Port : ActionPort  ActionType=then
  Call_Spi_AsyncTransmit : Subsystem
  Constant1 : Constant  OutDataTypeStr=boolean
  Constant2 : Constant  Value=0  OutDataTypeStr=uint8
  Constant3 : Constant  Value=0  OutDataTypeStr=boolean
  Constant4 : Constant  Value=0  OutDataTypeStr=boolean
  Constant5 : Constant  Value=SpiConf_SpiSequence_TmplMonrSeq1  OutDataTypeStr=uint8
  Constant6 : Constant  Value=SpiConf_SpiChannel_TmplMonrCh1  OutDataTypeStr=uint8
  Constant7 : Constant  Value=TMPLMONRSTSREG2READVAL_CNT_U16  OutDataTypeStr=uint16
  CopyRight1 : Subsystem  Description=|  mask(Copyright Information){none=on}
      | Copyright info block.                                               
      |                                                                     
      | Place copyright information at the top of every subsystem in design.
      mask prompts: none "No parameters"
      mask help: Place copyright information at the top of every subsystem in design.
      mask Display:
      | NxtrConf = 'Nexteer Confidential';
      | 
      | sys = bdroot; %handle for the current model ("system")
      | first = get_param(sys,'Created');
      | first = first(end-3:end);  %year is last four digits
      | 
      | last = get_param(sys,'LastModifiedDate');
      | if isempty(last)
      |     last = datestr(now,'yyyy');
      | else
      |     last = last(end-3:end);
      | end
      | 
      | if strcmp(first,last)
      |     fprintf('%s -- Copyright %s Nexteer',NxtrConf,first)
      | else
      |     fprintf('%s -- %s%s- %s Nexteer',NxtrConf,char(169),first,last)
      | end
  Data Store Write : DataStoreWrite  DataStoreName=TmplMonrSpiReadWrOrderFlg1
  Data Store Write2 : DataStoreWrite  DataStoreName=TmplMonrIninTestCmplFlg
      settings: AttributesFormatString=%<Name>
  Spi_WriteIB : Subsystem
  TmplMonrIninCntr : Outport
  TmplMonrIninTestCmpl : Outport  Port=2
  wires:
  Constant1/1 -> Data Store Write/1
  Constant5/1 -> Call_Spi_AsyncTransmit/1(Sequence)
  Constant6/1 -> Spi_WriteIB/1(Channel)
  Constant7/1 -> Spi_WriteIB/2(DataBufferPtr)
  Constant2/1 -> TmplMonrIninCntr/1
  Constant3/1 -> TmplMonrIninTestCmpl/1
  Constant4/1 -> Data Store Write2/1

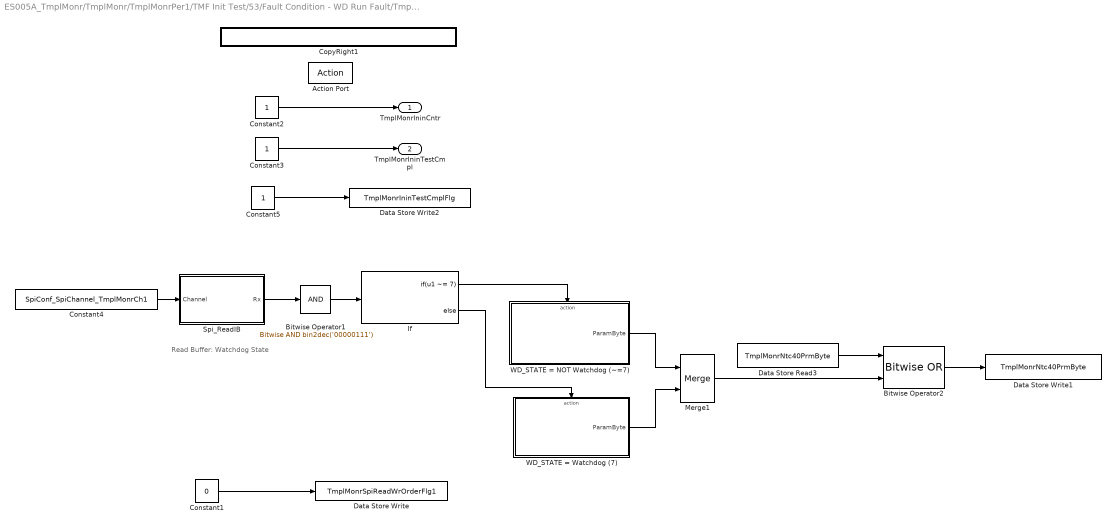
== system ES005A_TmplMonr/TmplMonr/TmplMonrPer1/TMF Init Test/53/Fault Condition - WD Run Fault/TmplMonrSpiReadWrOrderFlg1 = 1 (Read Buffer) ==
  note: Read Buffer: Watchdog State
  Action Port : ActionPort  ActionType=else
  Bitwise Operator1 : simulink/Logic and Bit Operations/Bitwise Operator  logicop=AND  UseBitMask=on  BitMask=bin2dec('00000111')  BitMaskRealWorld=Stored Integer
  Bitwise Operator2 : simulink/Logic and Bit Operations/Bitwise Operator  logicop=OR  UseBitMask=off  NumInputPorts=2  BitMask=bin2dec('00001111')  BitMaskRealWorld=Stored Integer
  Constant1 : Constant  Value=0  OutDataTypeStr=boolean
  Constant2 : Constant  OutDataTypeStr=uint8
  Constant3 : Constant  OutDataTypeStr=boolean
  Constant4 : Constant  Value=SpiConf_SpiChannel_TmplMonrCh1  OutDataTypeStr=uint8
  Constant5 : Constant  OutDataTypeStr=boolean
  CopyRight1 : Subsystem  Description=|  mask(Copyright Information){none=on}
      | Copyright info block.                                               
      |                                                                     
      | Place copyright information at the top of every subsystem in design.
      mask prompts: none "No parameters"
      mask help: Place copyright information at the top of every subsystem in design.
      mask Display:
      | NxtrConf = 'Nexteer Confidential';
      | 
      | sys = bdroot; %handle for the current model ("system")
      | first = get_param(sys,'Created');
      | first = first(end-3:end);  %year is last four digits
      | 
      | last = get_param(sys,'LastModifiedDate');
      | if isempty(last)
      |     last = datestr(now,'yyyy');
      | else
      |     last = last(end-3:end);
      | end
      | 
      | if strcmp(first,last)
      |     fprintf('%s -- Copyright %s Nexteer',NxtrConf,first)
      | else
      |     fprintf('%s -- %s%s- %s Nexteer',NxtrConf,char(169),first,last)
      | end
  Data Store Read3 : DataStoreRead  DataStoreName=TmplMonrNtc40PrmByte  DataStoreElements=TmplMonrNtc40PrmByte
  Data Store Write : DataStoreWrite  DataStoreName=TmplMonrSpiReadWrOrderFlg1
  Data Store Write1 : DataStoreWrite  DataStoreName=TmplMonrNtc40PrmByte
  Data Store Write2 : DataStoreWrite  DataStoreName=TmplMonrIninTestCmplFlg
      settings: AttributesFormatString=%<Name>
  If : If  IfExpression=u1 ~= 7
  Merge1 : Merge
  Spi_ReadIB : Subsystem
  WD_STATE = NOT Watchdog (~=7) : Subsystem  RequirementInfo={'linktype_rmi_doors' '0000c46a (/ESG Group/FDD Module Requirements/EA4 Specific/ES005A_TmplMonr)' '#ES005A_178' 'true' 'REQ: ES005A_178' '' } %GIDa_a99a9502_d42d_4074_927b_ce3461f07a7f
  WD_STATE = Watchdog (7) : Subsystem  RequirementInfo={'linktype_rmi_doors' '0000c46a (/ESG Group/FDD Module Requirements/EA4 Specific/ES005A_TmplMonr)' '#ES005A_175' 'true' 'REQ: ES005A_175' '' } %GIDa_7a1fb5a4_58f3_4f07_8ce4_3170f799d023
  TmplMonrIninCntr : Outport
  TmplMonrIninTestCmpl : Outport  Port=2
  wires:
  Constant1/1 -> Data Store Write/1
  Bitwise Operator1/1 -> If/1
  If/1 -> WD_STATE = NOT Watchdog (~=7)/Action
  If/2 -> WD_STATE = Watchdog (7)/Action
  Constant4/1 -> Spi_ReadIB/1(Channel)
  Spi_ReadIB/1(Rx) -> Bitwise Operator1/1
  Constant2/1 -> TmplMonrIninCntr/1
  WD_STATE = NOT Watchdog (~=7)/1(ParamByte) -> Merge1/1
  WD_STATE = Watchdog (7)/1(ParamByte) -> Merge1/2
  Constant3/1 -> TmplMonrIninTestCmpl/1
  Bitwise Operator2/1 -> Data Store Write1/1
  Data Store Read3/1 -> Bitwise Operator2/1
  Merge1/1 -> Bitwise Operator2/2
  Constant5/1 -> Data Store Write2/1

== system ES005A_TmplMonr/TmplMonr/TmplMonrPer1/TMF Init Test/53/IoHwAb_GetGpioPwrOutpEnaFb/CopyRight1 ==

== system ES005A_TmplMonr/TmplMonr/TmplMonrPer1/TMF Init Test/53/Normal Condition/CopyRight1 ==

== system ES005A_TmplMonr/TmplMonr/TmplMonrPer1/TMF Init Test/53/Set NTC 0x040 Note: Run last/FAILED = 1 ==
  note: NTCNR_0X040
      | Parameters:
      |     1 = 0000 0001 = Bit 0 = Fault Occured Between TmplMonrInitCntr =  10 ~ 11
      |     2 = 0000 0010 = Bit 1 = Fault Occured Between TmplMonrInitCntr = 13
      |     4 = 0000 0100 = Bit 2 = Fault Occured Between TmplMonrInitCntr = 15 ~ 16
      |     8 = 0000 1000 = Bit 3 = Fault Occured at TmplMonrInitCntr            = 18  (POE Fault)
      |   16 = 0001 0000 = Bit 4 = Fault Occured at TmplMonrInitCntr            = 19 (WD_STATE Fault)
      |   32 = 0010 0000 = Bit 5 = Fault Occured at TmplMonrInitCntr            = 21 (Edge/Valid Write Fault)
      |   64 = 0100 0000 = Bit 6 = Fault Occured at TmplMonrInitCntr            = 53 (POE + Non-WD Fault)
      | 128 = 1000 0000 = Bit 7 = Fault Occured at TmplMonrInitCntr            = 53 (POE + WD Fault)
  NtcStInfo : Inport  OutDataTypeStr=uint8
  Action Port : ActionPort  ActionType=else
  CopyRight1 : Subsystem  Description=|  mask(Copyright Information){none=on}
      | Copyright info block.                                               
      |                                                                     
      | Place copyright information at the top of every subsystem in design.
      mask prompts: none "No parameters"
      mask help: Place copyright information at the top of every subsystem in design.
      mask Display:
      | NxtrConf = 'Nexteer Confidential';
      | 
      | sys = bdroot; %handle for the current model ("system")
      | first = get_param(sys,'Created');
      | first = first(end-3:end);  %year is last four digits
      | 
      | last = get_param(sys,'LastModifiedDate');
      | if isempty(last)
      |     last = datestr(now,'yyyy');
      | else
      |     last = last(end-3:end);
      | end
      | 
      | if strcmp(first,last)
      |     fprintf('%s -- Copyright %s Nexteer',NxtrConf,first)
      | else
      |     fprintf('%s -- %s%s- %s Nexteer',NxtrConf,char(169),first,last)
      | end
  NTCFailStepCal - Non Debounce : Constant  Value=0  OutDataTypeStr=uint16
  NtcNr : Constant  Value=IninFlt
  NtcSts : Constant  OutDataTypeStr=uint8
  SetNtcSts : Subsystem
  wires:
  NtcNr/1 -> SetNtcSts/1(NtcNr)
  NTCFailStepCal - Non Debounce/1 -> SetNtcSts/4(DebStep)
  NtcSts/1 -> SetNtcSts/3(NtcSts)
  NtcStInfo/1 -> SetNtcSts/2(NtcStInfo)
